simulink model "Stepper_Model_Observer"  (R2017a)
settings: Solver=VariableStepAuto  StartTime=0.0  StopTime=60  RelTol=1e-3
values from neighbouring files (symbols this model uses):
  K = acker(A, B, [-10 -10 -10])    [Simulation_main.m]
  Ptheta0 = 0    [Simulation_main.m]
  stepInput = 0    [Simulation_main.m]
libraries: simulink x2
settings Model: Creator=Patrick  LastModifiedBy=Patrick

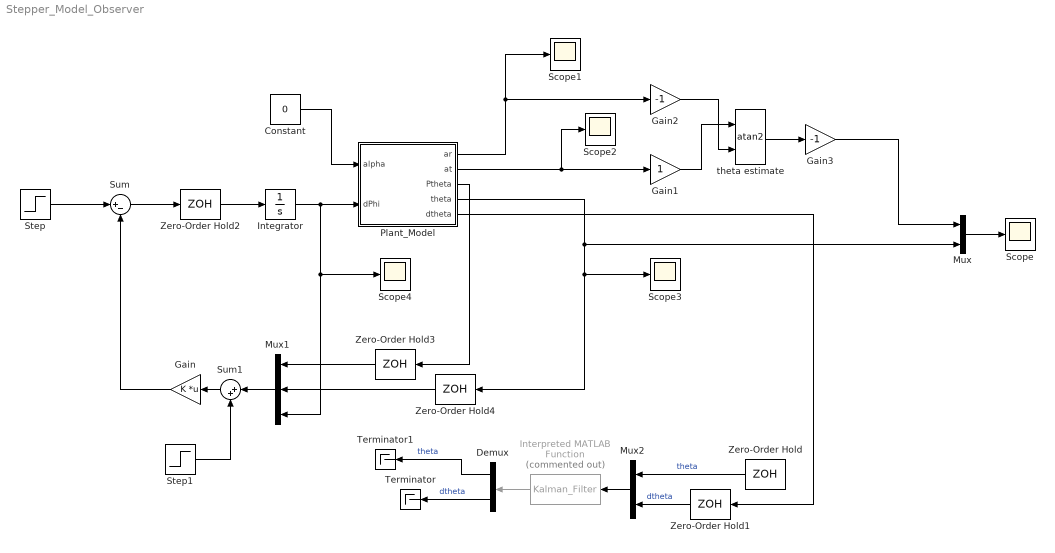
== system Stepper_Model_Observer ==
  Constant : Constant  Value=0
  Demux : Demux  Outputs=2
  Gain : Gain  Gain=K  Multiplication=Matrix(K*u)
  Gain1 : Gain
  Gain2 : Gain  Gain=-1
  Gain3 : Gain  Gain=-1
  Integrator : Integrator
  Interpreted MATLAB Function : MATLABFcn  Commented=on  MATLABFcn=Kalman_Filter  OutputDimensions=[2 1]  Output1D=off
  Mux : Mux  Inputs=2
  Mux1 : Mux  Inputs=3
  Mux2 : Mux  Inputs=2
  Plant_Model : Subsystem
  Scope{,1..4} (5 alike) : Scope
  Step : Step  Time=10  After=stepInput  SampleTime=0
  Step1 : Step  Time=10  After=0  SampleTime=0
  Sum : Sum  Inputs=|+-
  Sum1 : Sum  Inputs=|++
  Terminator : Terminator
  Terminator1 : Terminator
  Zero-Order Hold{,1..4} (5 alike) : ZeroOrderHold  SampleTime=0.01
  theta estimate : Trigonometry  Operator=atan2  OutputSignalType=real
  wires:
  Constant/1 -> Plant_Model/1("alpha ")
  Mux/1 -> Scope/1
  Step/1 -> Sum/1
  Plant_Model/4(theta) -> Scope3/1, Zero-Order Hold4/1, Mux/2
  Zero-Order Hold/1 -> Mux2/1  "theta"
  Zero-Order Hold1/1 -> Mux2/2  "dtheta"
  Plant_Model/5(dtheta) -> Zero-Order Hold1/1
  Demux/2 -> Terminator/1  "dtheta"
  Sum/1 -> Zero-Order Hold2/1
  Mux2/1 -> Interpreted MATLAB Function/1
  Interpreted MATLAB Function/1 -> Demux/1
  Plant_Model/1(ar) -> Gain2/1, Scope1/1
  Plant_Model/2(at) -> Scope2/1, Gain1/1
  Demux/1 -> Terminator1/1  "theta"
  Gain/1 -> Sum/2
  Gain1/1 -> theta estimate/1
  Gain2/1 -> theta estimate/2
  Zero-Order Hold3/1 -> Mux1/1
  Zero-Order Hold4/1 -> Mux1/2
  Zero-Order Hold2/1 -> Integrator/1
  Integrator/1 -> Mux1/3, Scope4/1, Plant_Model/2(dPhi)
  Plant_Model/3(Ptheta) -> Zero-Order Hold3/1
  Sum1/1 -> Gain/1
  Mux1/1 -> Sum1/1
  Step1/1 -> Sum1/2
  theta estimate/1 -> Gain3/1
  Gain3/1 -> Mux/1

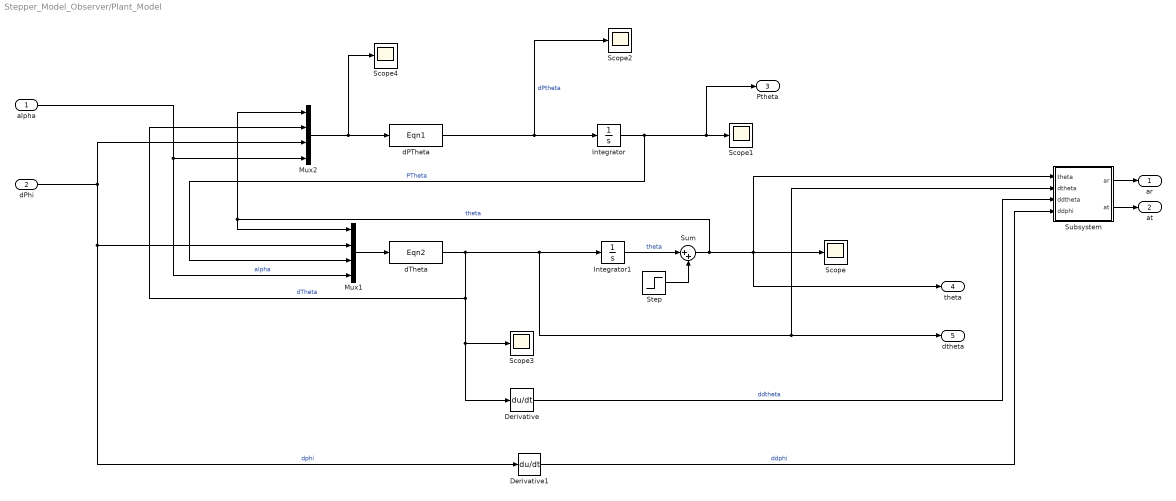
== system Stepper_Model_Observer/Plant_Model ==
  "alpha " : Inport
  dPhi : Inport  Port=2
  Derivative : Derivative
  Derivative1 : Derivative
  Integrator : Integrator  InitialCondition=Ptheta0
  Integrator1 : Integrator  InitialCondition=0.1
  Mux1 : Mux  Inputs=[1 1 1 1]
  Mux2 : Mux  Inputs=[1 1 1 1]
  Scope{,1..4} (5 alike) : Scope
  Step : Step  Time=10  After=.1  SampleTime=0
  Subsystem : Subsystem
  Sum : Sum  Inputs=|++
  dPTheta : MATLABFcn  MATLABFcn=Eqn1  OutputDimensions=[1 1]  Output1D=off
  dTheta : MATLABFcn  MATLABFcn=Eqn2  OutputDimensions=[1 1]  Output1D=off
  ar : Outport  PortDimensions=[1 1]
  at : Outport  Port=2  PortDimensions=[1 1]
  Ptheta : Outport  Port=3  PortDimensions=[1 1]
  theta : Outport  Port=4  PortDimensions=[1 1]
  dtheta : Outport  Port=5  PortDimensions=[1 1]
  wires:
  Integrator/1 -> Ptheta/1, Scope1/1, Mux1/3  "PTheta"
  dPhi/1 -> Mux2/3, Derivative1/1, Mux1/2  "dphi"
  dPTheta/1 -> Integrator/1, Scope2/1  "dPtheta"
  dTheta/1 -> Derivative/1, Scope3/1, Mux2/2, Subsystem/2(dtheta), dtheta/1, Integrator1/1  "dTheta"
  Mux2/1 -> Scope4/1, dPTheta/1
  Mux1/1 -> dTheta/1
  "alpha "/1 -> Mux1/4, Mux2/4  "alpha"
  Derivative/1 -> Subsystem/3(ddtheta)  "ddtheta"
  Derivative1/1 -> Subsystem/4(ddphi)  "ddphi"
  Subsystem/1(ar) -> ar/1
  Subsystem/2(at) -> at/1
  Sum/1 -> Mux2/1, Mux1/1, Subsystem/1(theta), theta/1, Scope/1  "theta"
  Integrator1/1 -> Sum/1  "theta"
  Step/1 -> Sum/2

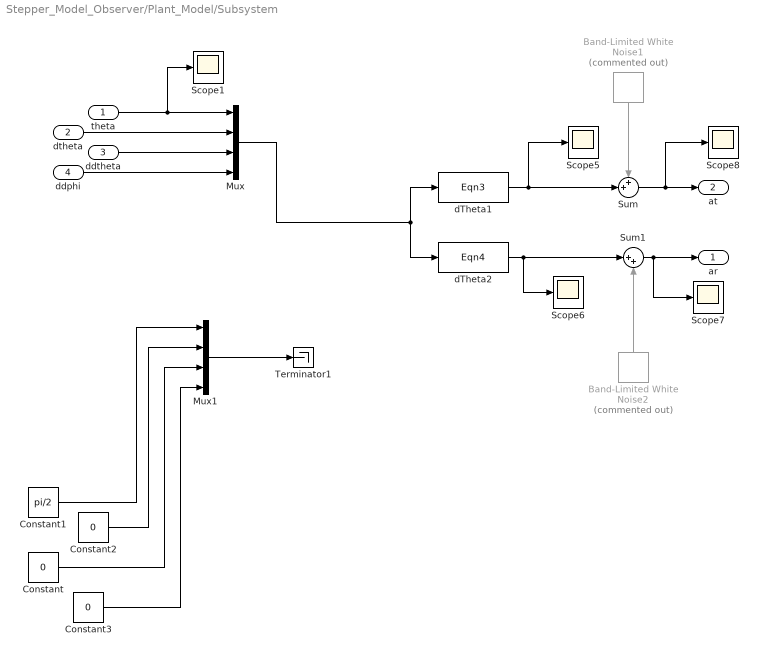
== system Stepper_Model_Observer/Plant_Model/Subsystem ==
  theta : Inport
  dtheta : Inport  Port=2
  ddtheta : Inport  Port=3
  ddphi : Inport  Port=4
  Band-Limited White Noise1 : simulink/Sources/Band-Limited White Noise  Commented=on  Cov=[0.00001]  Ts=.01  seed=[23341]
  Band-Limited White Noise2 : simulink/Sources/Band-Limited White Noise  Commented=on  Cov=[0.00001]  Ts=.01  seed=[23341]
  Constant : Constant  Value=0
  Constant1 : Constant  Value=pi/2
  Constant2 : Constant  Value=0
  Constant3 : Constant  Value=0
  Mux : Mux
  Mux1 : Mux
  Scope{1,5..8} (5 alike) : Scope
  Sum : Sum  Inputs=++|
  Sum1 : Sum  Inputs=|++
  Terminator1 : Terminator
  dTheta1 : MATLABFcn  MATLABFcn=Eqn3  OutputDimensions=[1 1]  Output1D=off
  dTheta2 : MATLABFcn  MATLABFcn=Eqn4  OutputDimensions=[1 1]  Output1D=off
  ar : Outport  PortDimensions=[1 1]
  at : Outport  Port=2  PortDimensions=[1 1]
  wires:
  theta/1 -> Scope1/1, Mux/1
  dtheta/1 -> Mux/2
  Mux/1 -> dTheta1/1, dTheta2/1
  Sum/1 -> at/1, Scope8/1
  dTheta2/1 -> Sum1/1, Scope6/1
  Sum1/1 -> ar/1, Scope7/1
  dTheta1/1 -> Sum/2, Scope5/1
  ddphi/1 -> Mux/4
  ddtheta/1 -> Mux/3
  Band-Limited White Noise1/1 -> Sum/1
  Band-Limited White Noise2/1 -> Sum1/2
  Constant3/1 -> Mux1/4
  Constant1/1 -> Mux1/1
  Constant2/1 -> Mux1/2
  Constant/1 -> Mux1/3
  Mux1/1 -> Terminator1/1
